simulink model "P_like"  (R2015b)
settings: Solver=VariableStepAuto  StartTime=0.0  StopTime=100  RelTol=1e-3
undefined symbols (not defined in the file or in its folder): Dm, Ds, Kdp, Kpp
settings Model: Creator=TOSHIBA  LastModifiedBy=TOSHIBA

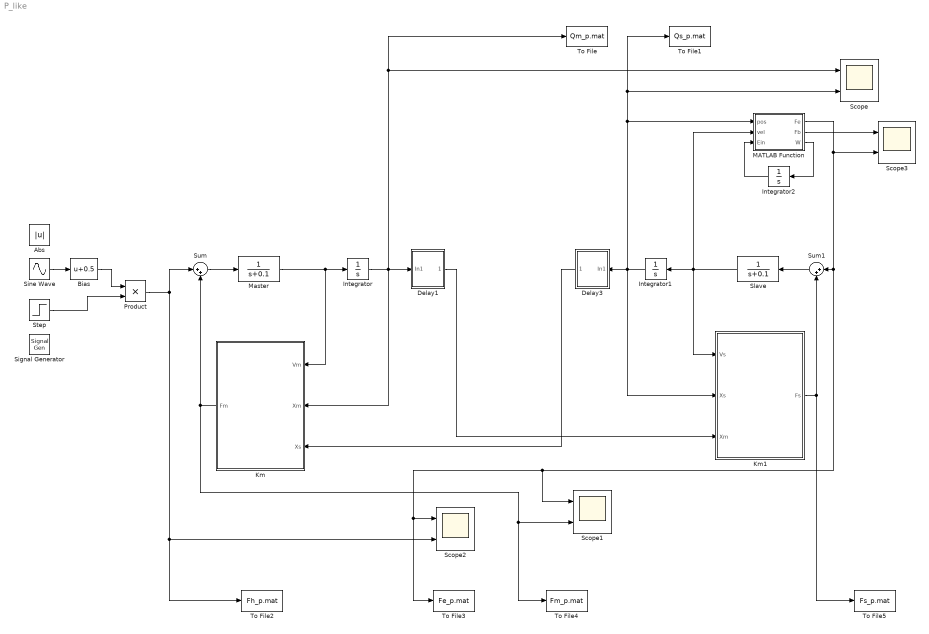
== system P_like ==
  Abs : Abs
  Bias : Bias  Bias=0.5
  Delay1 : Subsystem
  Delay3 : Subsystem
  Integrator : Integrator
  Integrator1 : Integrator
  Integrator2 : Integrator
  Km : Subsystem
  Km1 : Subsystem
  MATLAB Function : MATLAB Function  TreatAsAtomicUnit=on
  Master : TransferFcn  Denominator=[1 0.1]
  Product : Product
  Scope{,1..3} (4 alike) : Scope  NumInputPorts=2
  Signal Generator : SignalGenerator  WaveForm=square  Amplitude=-1  Frequency=0.05*pi  Units=rad/sec
  Sine Wave : Sin  Frequency=pi/20  SampleTime=0
  Slave : TransferFcn  Denominator=[1 0.1]
  Step : Step  Time=100  Before=1  After=0  SampleTime=0
  Sum : Sum  Inputs=|++
  Sum1 : Sum  Inputs=|++
  To File : ToFile  Filename=Qm_p.mat  MatrixName=Qm_p  SaveFormat=Timeseries
  To File1 : ToFile  Filename=Qs_p.mat  MatrixName=Qs_p  SaveFormat=Timeseries
  To File2 : ToFile  Filename=Fh_p.mat  MatrixName=Fh_p  SaveFormat=Timeseries
  To File3 : ToFile  Filename=Fe_p.mat  MatrixName=Fe_p  SaveFormat=Timeseries
  To File4 : ToFile  Filename=Fm_p.mat  MatrixName=Fm_p  SaveFormat=Timeseries
  To File5 : ToFile  Filename=Fs_p.mat  MatrixName=Fs_p  SaveFormat=Timeseries
  wires:
  Sum/1 -> Master/1
  Master/1 -> Km/1(Vm), Integrator/1
  Integrator/1 -> Delay1/1(In1), Km/2(Xm), To File/1, Scope/1
  Km/1(Fm) -> Sum/2, To File4/1, Scope1/2
  Slave/1 -> MATLAB Function/2(vel), Km1/1(Vs), Integrator1/1
  Km1/1(Fs) -> To File5/1, Sum1/2
  Sum1/1 -> Slave/1
  Delay1/1(Out1) -> Km1/3(Xm)
  Delay3/1(Out1) -> Km/3(Xs)
  Integrator1/1 -> Delay3/1(In1), MATLAB Function/1(pos), To File1/1, Scope/2, Km1/2(Xs)
  MATLAB Function/1(Fe) -> Scope1/1, To File3/1, Scope2/1, Sum1/1, Scope3/2
  MATLAB Function/3(W) -> Integrator2/1
  Integrator2/1 -> MATLAB Function/3(Ein)
  MATLAB Function/2(Fb) -> Scope3/1
  Sine Wave/1 -> Bias/1
  Bias/1 -> Product/1
  Product/1 -> To File2/1, Scope2/2, Sum/1
  Step/1 -> Product/2

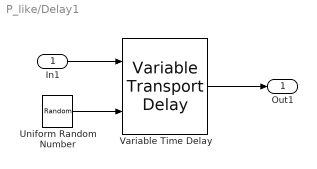
== system P_like/Delay1 ==
  In1 : Inport
  Uniform Random Number : UniformRandomNumber  Minimum=0  Maximum=Dm  SampleTime=0.1
  Variable Time Delay : VariableTransportDelay  MaximumDelay=Dm
  Out1 : Outport
  wires:
  Variable Time Delay/1 -> Out1/1
  In1/1 -> Variable Time Delay/1
  Uniform Random Number/1 -> Variable Time Delay/2

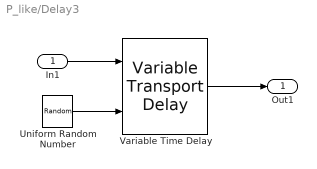
== system P_like/Delay3 ==
  In1 : Inport
  Uniform Random Number : UniformRandomNumber  Minimum=0  Maximum=Ds  SampleTime=0.1
  Variable Time Delay : VariableTransportDelay  MaximumDelay=Ds
  Out1 : Outport
  wires:
  Uniform Random Number/1 -> Variable Time Delay/2
  In1/1 -> Variable Time Delay/1
  Variable Time Delay/1 -> Out1/1

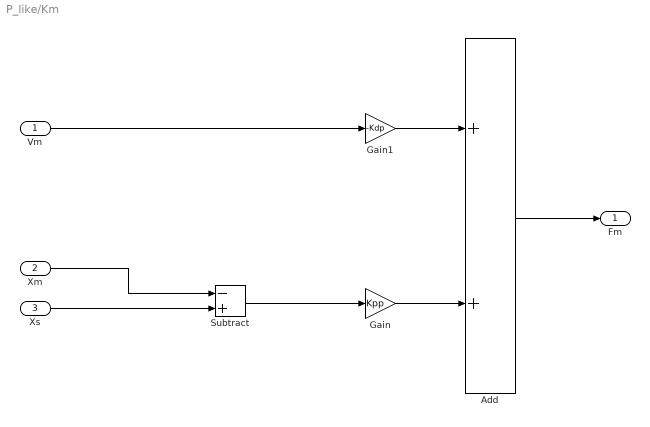
== system P_like/Km ==
  Vm : Inport
  Xm : Inport  Port=2
  Xs : Inport  Port=3
  Add : Sum
  Gain : Gain  Gain=Kpp
  Gain1 : Gain  Gain=-Kdp
  Subtract : Sum  Inputs=-+
  Fm : Outport
  wires:
  Xm/1 -> Subtract/1
  Xs/1 -> Subtract/2
  Gain/1 -> Add/2
  Gain1/1 -> Add/1
  Add/1 -> Fm/1
  Vm/1 -> Gain1/1
  Subtract/1 -> Gain/1

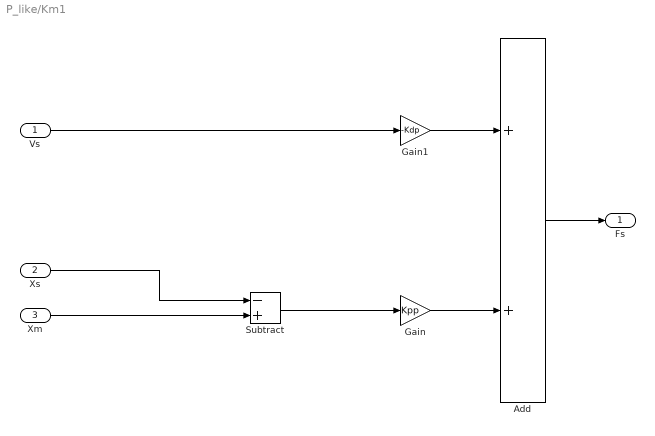
== system P_like/Km1 ==
  Vs : Inport
  Xs : Inport  Port=2
  Xm : Inport  Port=3
  Add : Sum
  Gain : Gain  Gain=Kpp
  Gain1 : Gain  Gain=-Kdp
  Subtract : Sum  Inputs=-+
  Fs : Outport
  wires:
  Xs/1 -> Subtract/1
  Xm/1 -> Subtract/2
  Subtract/1 -> Gain/1
  Vs/1 -> Gain1/1
  Gain/1 -> Add/2
  Gain1/1 -> Add/1
  Add/1 -> Fs/1

== matlab function P_like/MATLAB Function ==
  data: pos input; vel input; Fe output; Fb output; Ein input; W output
function [Fe, Fb, W] = Envir(pos,vel,Ein)
%#codegen
kWall = 10000;
bWall = 0;
if pos>=0.5
    Fk=-(pos-0.5)*kWall;
    if Ein<=10
        Fb=bWall*vel;
    else
        Fb=0;
    end
    Fe=Fk+Fb;
    W=Fb*vel;
else
    Fe=0;
    Fb=0;
    W=0;
end
